simulink subsystem "encoders"  (R2023b)
settings: Solver=VariableStepAuto  StartTime=0.0  StopTime=10.0  RelTol=1e-3
libraries: arduinosensorlib x2
settings Model: Creator=Carlos  LastModifiedBy=Carlos

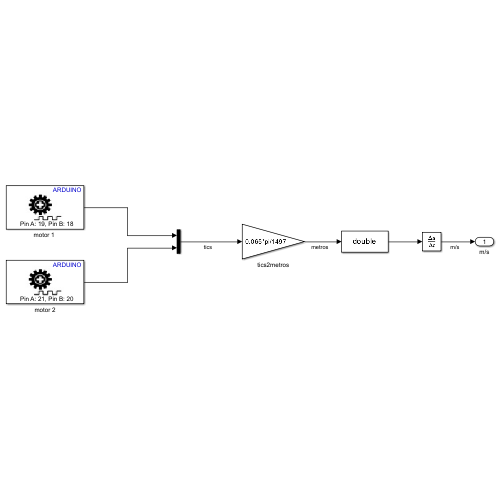
[thumbnail: Simulink's stored preview of the top-level diagram]
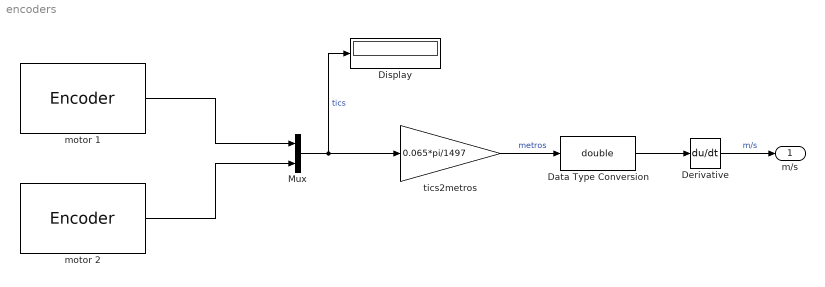
== system encoders ==
  Data Type Conversion : DataTypeConversion  OutDataTypeStr=double  SaturateOnIntegerOverflow=off  RndMeth=Floor
  Derivative : Derivative
  Display : Display
  Mux : Mux  Inputs=2
  "motor 1 " : arduinosensorlib/Encoder  InputA=18  InputB=19  Mode=No reset  SampleTime=-1
  motor 2 : arduinosensorlib/Encoder  InputA=21  InputB=20  Mode=No reset  SampleTime=-1
  tics2metros : Gain  Gain=0.065*pi/1497
  m/s : Outport
  wires:
  tics2metros/1 -> Data Type Conversion/1  "metros"
  "motor 1 "/1 -> Mux/1
  Data Type Conversion/1 -> Derivative/1
  Mux/1 -> tics2metros/1, Display/1  "tics"
  motor 2/1 -> Mux/2
  Derivative/1 -> m/s/1  "m/s"
